simulink model "BugE_v0_40_MAS"  (R2015b)
settings: Solver=FixedStepDiscrete  StartTime=0.0  StopTime=inf  FixedStep=sample_time  RelTol=1e-3
values from neighbouring files (symbols this model uses):
  AB_diode_dV = 0.9    [main_sync.m]
  air_density = 1.225    [main_sync.m]
  bus_charger_Pmax = 1000    [main_sync.m]
  bus_load_Pmax_abs = 500    [main_sync.m]
  capInitVolt = capVmax*sqrt(capInitSoC)    [main_sync.m]
  cyc_kph = [cyc_kph(:,1), cyc_kph(:,2)*speed_max_limit/speed_max]    [main_sync.m]
  cyc_repeat = 0    [main_sync.m]
  ess1_init_soc = 1    [main_sync.m]
  ess1_soh = 1    [main_sync.m]
  ess2_init_soc = 1    [main_sync.m]
  ess2_soh = 1    [main_sync.m]
  ess3_init_soc = 1    [main_sync.m]
  ess3_soh = 1    [main_sync.m]
  ess4_init_soc = 1    [main_sync.m]
  ess4_soh = 1    [main_sync.m]
  ess5_init_soc = 1    [main_sync.m]
  ess5_soh = 1    [main_sync.m]
  gear_ratio = 6    [main_sync.m]
  loadpower = rawcsv(:,2)    [main_sync.m]
  loadtime = rawcsv(:,1)    [main_sync.m]
  lockSOCs = 0    [main_sync.m]
  max_brk_torque = 300    [main_sync.m]
  no_wheels = 3    [main_sync.m]
  period2 = max(loadtime)    [main_sync.m]
  PV_Pmax = 100    [main_sync.m]
  sample_time = 0.01    [main_sync.m]
  startup_seq_step_delay = 0.2    [main_sync.m]
  stop_option = 0    [main_sync.m]
  use_drive_cycle = 1    [main_sync.m]
  use_real_subs_loads = 1    [main_sync.m]
  vbus_max = 25    [main_sync.m]
  vbus_min = 17    [main_sync.m]
  vbus_safety_threshold = 2    [main_sync.m]
  vbus_threshold = 20    [main_sync.m]
  veh_CD = 0.35    [main_sync.m]
  veh_FA = 1.543    [main_sync.m]
  veh_gravity = 9.81*veh_mass    (= 1863.9)    [main_sync.m]
  veh_mass = 190    [main_sync.m]
  wh_1st_rrc = 0.02    [main_sync.m]
  wh_bearing_frc = 0.0015    [main_sync.m]
  wh_inertia = 0.0556    [main_sync.m]
  wh_radius = 0.508/2    (= 0.254)    [main_sync.m]
undefined symbols (not defined in the file or in its folder): capC, capR, cyc_acc, cyc_avg_time_samples, cyc_brk, cyc_grade, cyc_key, DCM_eff_factor_for_Vin, DCM_eff_for_Iout, DCM_Iout, DCM_Iout_max, DCM_Pin_noload, DCM_Pout_max, DCM_Vin, DCM_Vout, DiscIntNeverNeededParam, ess2_coulombic_eff, ess2_Ineg_max_SOC, ess2_Ineg_max_temp, ess2_Ipos_max_SOC, ess2_Ipos_max_temp, ess2_max_ah_cap, ess2_max_volts, ess2_min_volts, ess2_module_parallel, ess2_module_series, ess2_r_dis, ess2_soc, ess2_SOC_for_Ilimit, ess2_temp_for_Ilimit, ess2_temp_max, ess2_tmp, ess2_voc, ess3_coulombic_eff, ess3_max_ah_cap, ess3_module_parallel, ess3_module_series, ess3_r_dis, ess3_soc, ess3_tmp, ess3_voc, ess_coulombic_eff, ess_Ineg_max_SOC, ess_Ineg_max_temp, ess_Ipos_max_SOC, ess_Ipos_max_temp, ess_max_ah_cap, ess_max_volts, ess_min_volts, ess_module_parallel, ess_module_series, ess_nominal_volts, ess_r_dis, ess_soc, ess_SOC_for_Ilimit, ess_temp_for_Ilimit, ess_temp_max, ess_tmp, ess_voc, MC_eff1 ... (+17)
libraries: simulink x139, commfilt2 x1, simulink_extras x1
(part 7 of 7)

== system BugE_v0_40_MAS/Master Controller/Operating Mode Controller/State machine 0 std, 1 startup, 2 acc, 3 drv, 4 fault/pass10 ==
  I : Inport
  Logical Operator : Logic  Operator=NOT  AllPortsSameDT=off  OutDataTypeStr=boolean
  Logical Operator1 : Logic  Operator=NOT  AllPortsSameDT=off  OutDataTypeStr=boolean
  O : Outport
  wires:
  I/1 -> Logical Operator/1
  Logical Operator1/1 -> O/1
  Logical Operator/1 -> Logical Operator1/1

== system BugE_v0_40_MAS/Master Controller/Operating Mode Controller/State machine 0 std, 1 startup, 2 acc, 3 drv, 4 fault/pass2 ==
  I : Inport
  Logical Operator : Logic  Operator=NOT  AllPortsSameDT=off  OutDataTypeStr=boolean
  Logical Operator1 : Logic  Operator=NOT  AllPortsSameDT=off  OutDataTypeStr=boolean
  O : Outport
  wires:
  I/1 -> Logical Operator/1
  Logical Operator1/1 -> O/1
  Logical Operator/1 -> Logical Operator1/1

== system BugE_v0_40_MAS/Master Controller/Operating Mode Controller/State machine 0 std, 1 startup, 2 acc, 3 drv, 4 fault/pass3 ==
  I : Inport
  Logical Operator : Logic  Operator=NOT  AllPortsSameDT=off  OutDataTypeStr=boolean
  Logical Operator1 : Logic  Operator=NOT  AllPortsSameDT=off  OutDataTypeStr=boolean
  O : Outport
  wires:
  I/1 -> Logical Operator/1
  Logical Operator1/1 -> O/1
  Logical Operator/1 -> Logical Operator1/1

== system BugE_v0_40_MAS/Master Controller/Operating Mode Controller/State machine 0 std, 1 startup, 2 acc, 3 drv, 4 fault/pass4 ==
  I : Inport
  Logical Operator : Logic  Operator=NOT  AllPortsSameDT=off  OutDataTypeStr=boolean
  Logical Operator1 : Logic  Operator=NOT  AllPortsSameDT=off  OutDataTypeStr=boolean
  O : Outport
  wires:
  I/1 -> Logical Operator/1
  Logical Operator1/1 -> O/1
  Logical Operator/1 -> Logical Operator1/1

== system BugE_v0_40_MAS/Master Controller/Operating Mode Controller/State machine 0 std, 1 startup, 2 acc, 3 drv, 4 fault/pass5 ==
  I : Inport
  Logical Operator : Logic  Operator=NOT  AllPortsSameDT=off  OutDataTypeStr=boolean
  Logical Operator1 : Logic  Operator=NOT  AllPortsSameDT=off  OutDataTypeStr=boolean
  O : Outport
  wires:
  I/1 -> Logical Operator/1
  Logical Operator1/1 -> O/1
  Logical Operator/1 -> Logical Operator1/1

== system BugE_v0_40_MAS/Master Controller/Secondary Objectives/MB SOC balancing/Balancing type: 1: none, 2: P>0, 3: P<0 ==
  enable : Inport
  DCDC Iout (bus side) : Inport  Port=2
  enabled MODs : Inport  Port=3
  Data Type Conversion : DataTypeConversion
  Dead Zone +- 10E-3 : DeadZone  LowerValue=-10E-3  UpperValue=10E-3  SaturateOnIntegerOverflow=on
  Iout_total MB DCDC : Sum  Inputs=+
  Mux3 : Mux  Inputs=3
  P<0 : Gain  Gain=3  OutDataTypeStr=double
  P<0 balancing : simulink/Logic and Bit Operations/Compare To Constant  relop=<  const=0  OutDataTypeStr=boolean
  P=0 : Gain  OutDataTypeStr=double
  P>0 : Gain  Gain=2  OutDataTypeStr=double
  P>0 balancing : simulink/Logic and Bit Operations/Compare To Constant  relop=>  const=0  OutDataTypeStr=boolean
  Product : Product
  Saturation : Saturate  UpperLimit=3  LowerLimit=1
  and : Logic  AllPortsSameDT=off  OutDataTypeStr=boolean
  enable balancing : simulink/Logic and Bit Operations/Compare To Constant  relop=>=  const=2  OutDataTypeStr=boolean
  max : MinMax  Function=max
  no balancing : simulink/Logic and Bit Operations/Compare To Constant  relop===  const=0  OutDataTypeStr=boolean
  sum : Sum  Inputs=+
  type : Outport
  wires:
  no balancing/1 -> P=0/1
  DCDC Iout (bus side)/1 -> Iout_total MB DCDC/1
  Mux3/1 -> max/1
  Dead Zone +- 10E-3/1 -> no balancing/1, P<0 balancing/1, P>0 balancing/1
  P<0 balancing/1 -> P<0/1
  P>0/1 -> Mux3/2
  P<0/1 -> Mux3/3
  Iout_total MB DCDC/1 -> Dead Zone +- 10E-3/1
  P=0/1 -> Mux3/1
  P>0 balancing/1 -> P>0/1
  Product/1 -> Saturation/1
  max/1 -> Product/2
  enable/1 -> and/1
  Data Type Conversion/1 -> Product/1
  Saturation/1 -> type/1
  enabled MODs/1 -> sum/1
  sum/1 -> enable balancing/1
  enable balancing/1 -> and/2
  and/1 -> Data Type Conversion/1

== system BugE_v0_40_MAS/Master Controller/Secondary Objectives/MB SOC balancing/MB balancing through load distribution ==
  note: Pout MB DCDC
      | 1: none, 2: P>0, 3: P<0
  distribution type : Inport
  MOD's EN : Inport  Port=2
  MB SOCs : Inport  Port=3
  1/rel SOCs : Switch  Criteria=u2 > Threshold
  1/u : Math  Operator=reciprocal  RndMeth=Zero  SaturateOnIntegerOverflow=on
  >= eps : Saturate  UpperLimit=inf  LowerLimit=eps
  Constant1 : Constant  Value=3  SampleTime=sample_time
  Multiport Switch2 : MultiPortSwitch  SaturateOnIntegerOverflow=on
  SOCmax : MinMax  Function=max
  Scope : Scope
  "[1,10]" : Saturate  UpperLimit=10  LowerLimit=1
  "[eps,1]" : Saturate  UpperLimit=1  LowerLimit=eps
  bool2dbl : DataTypeConversion  OutDataTypeStr=double
  filtered SOCs (0 for dsbl'ed) : Product
  normalize (smallest = 1) : Product  Inputs=*/
  ones : Subsystem
  positive min : Subsystem
  relative SOCs : Product  Inputs=*/
  strengthen ratios : Math  Operator=pow  SaturateOnIntegerOverflow=on
  MB slope adj : Outport
  wires:
  distribution type/1 -> Multiport Switch2/1
  MOD's EN/1 -> bool2dbl/1
  bool2dbl/1 -> filtered SOCs (0 for dsbl'ed)/2
  MB SOCs/1 -> filtered SOCs (0 for dsbl'ed)/1
  "[eps,1]"/1 -> 1/u/1
  >= eps/1 -> relative SOCs/2
  SOCmax/1 -> >= eps/1
  filtered SOCs (0 for dsbl'ed)/1 -> 1/rel SOCs/2, SOCmax/1, relative SOCs/1, ones/1(I)
  1/u/1 -> 1/rel SOCs/1
  ones/1(O) -> 1/rel SOCs/3, Multiport Switch2/2
  relative SOCs/1 -> "[eps,1]"/1, Multiport Switch2/3
  Constant1/1 -> strengthen ratios/2
  1/rel SOCs/1 -> Multiport Switch2/4
  positive min/1(O) -> normalize (smallest = 1)/2
  Multiport Switch2/1 -> normalize (smallest = 1)/1, positive min/1(I)
  normalize (smallest = 1)/1 -> Scope/1, strengthen ratios/1
  strengthen ratios/1 -> "[1,10]"/1
  "[1,10]"/1 -> MB slope adj/1

== system BugE_v0_40_MAS/Master Controller/Secondary Objectives/Motor MBDCDC boost/ones ==
  I : Inport
  Bias : Bias  Bias=1
  Gain : Gain  Gain=0
  bool2dbl : DataTypeConversion  OutDataTypeStr=double
  O : Outport
  wires:
  Bias/1 -> O/1
  I/1 -> bool2dbl/1
  Gain/1 -> Bias/1
  bool2dbl/1 -> Gain/1

== system BugE_v0_40_MAS/Master Controller/System Health/Internally detected faults/20s moving avg (1//20 samples)1 ==
  In1 : Inport
  Counter Limited : simulink/Sources/Counter Limited  uplimit=19  tsamp=sample_time
  Triggered Subsystem : Subsystem  TreatAsAtomicUnit=on
  Out1 : Outport
  wires:
  Triggered Subsystem/1(Out1) -> Out1/1
  Counter Limited/1 -> Triggered Subsystem/Trigger
  In1/1 -> Triggered Subsystem/1(In1)

== system BugE_v0_40_MAS/Master Controller/System Health/Internally detected faults/20s moving avg (1//20 samples)3 ==
  In1 : Inport
  Counter Limited : simulink/Sources/Counter Limited  uplimit=19  tsamp=sample_time
  Triggered Subsystem : Subsystem  TreatAsAtomicUnit=on
  Out1 : Outport
  wires:
  Triggered Subsystem/1(Out1) -> Out1/1
  Counter Limited/1 -> Triggered Subsystem/Trigger
  In1/1 -> Triggered Subsystem/1(In1)

== system BugE_v0_40_MAS/Master Controller/System Health/Internally detected faults/40s moving avg (1//40 samples) ==
  In1 : Inport
  Counter Limited : simulink/Sources/Counter Limited  uplimit=39  tsamp=sample_time
  Triggered Subsystem : Subsystem  TreatAsAtomicUnit=on
  Out1 : Outport
  wires:
  Triggered Subsystem/1(Out1) -> Out1/1
  Counter Limited/1 -> Triggered Subsystem/Trigger
  In1/1 -> Triggered Subsystem/1(In1)

== system BugE_v0_40_MAS/Master Controller/System Health/Internally detected faults/diff >= 10% (or >1W for cmd=0) ==
  command : Inport
  result : Inport  Port=2
  !=0 : simulink/Logic and Bit Operations/Compare To Zero  relop=~=  OutDataTypeStr=boolean
  Constant : Constant  SampleTime=sample_time
  "Dead Zone [-0.1, 0.1]" : DeadZone  LowerValue=-0.1  UpperValue=0.1  SaturateOnIntegerOverflow=on
  "Dead Zone [-1, 1]" : DeadZone  LowerValue=-1  UpperValue=1  SaturateOnIntegerOverflow=on
  Divide : Product  Inputs=*/
  Subtract : Sum  Inputs=-+
  Switch avoid 0 div : Switch  Criteria=u2 > Threshold
  case where cmd=0 : Switch  Criteria=u2 > Threshold
  ~=0 : simulink/Logic and Bit Operations/Compare To Zero  relop=~=  OutDataTypeStr=boolean
  significant diff detected : Outport
  wires:
  Subtract/1 -> Divide/1
  command/1 -> !=0/1, Switch avoid 0 div/1, Subtract/2
  Divide/1 -> "Dead Zone [-0.1, 0.1]"/1
  ~=0/1 -> significant diff detected/1
  "Dead Zone [-0.1, 0.1]"/1 -> case where cmd=0/1
  Constant/1 -> Switch avoid 0 div/3
  Switch avoid 0 div/1 -> Divide/2
  !=0/1 -> case where cmd=0/2, Switch avoid 0 div/2
  result/1 -> "Dead Zone [-1, 1]"/1, Subtract/1
  "Dead Zone [-1, 1]"/1 -> case where cmd=0/3
  case where cmd=0/1 -> ~=0/1

== system BugE_v0_40_MAS/Master Controller/System Health/Internally detected faults/diff >= 10% (or >1W for cmd=0)1 ==
  command : Inport
  result : Inport  Port=2
  !=0 : simulink/Logic and Bit Operations/Compare To Zero  relop=~=  OutDataTypeStr=boolean
  Constant : Constant  SampleTime=sample_time
  "Dead Zone [-0.1, 0.1]" : DeadZone  LowerValue=-0.1  UpperValue=0.1  SaturateOnIntegerOverflow=on
  "Dead Zone [-1, 1]" : DeadZone  LowerValue=-1  UpperValue=1  SaturateOnIntegerOverflow=on
  Divide : Product  Inputs=*/
  Subtract : Sum  Inputs=-+
  Switch avoid 0 div : Switch  Criteria=u2 > Threshold
  case where cmd=0 : Switch  Criteria=u2 > Threshold
  ~=0 : simulink/Logic and Bit Operations/Compare To Zero  relop=~=  OutDataTypeStr=boolean
  significant diff detected : Outport
  wires:
  Subtract/1 -> Divide/1
  command/1 -> !=0/1, Switch avoid 0 div/1, Subtract/2
  Divide/1 -> "Dead Zone [-0.1, 0.1]"/1
  ~=0/1 -> significant diff detected/1
  "Dead Zone [-0.1, 0.1]"/1 -> case where cmd=0/1
  Constant/1 -> Switch avoid 0 div/3
  Switch avoid 0 div/1 -> Divide/2
  !=0/1 -> case where cmd=0/2, Switch avoid 0 div/2
  result/1 -> "Dead Zone [-1, 1]"/1, Subtract/1
  "Dead Zone [-1, 1]"/1 -> case where cmd=0/3
  case where cmd=0/1 -> ~=0/1

== system BugE_v0_40_MAS/Misc/Energy Calculations/E_battery_total/Battery losses ==
  Add : Sum  Inputs=5
  Unit Delay : UnitDelay  SampleTime=-1
  Out1 : Outport
  wires:
  [E_batt_loss2] -> Add/2
  [E_batt_loss1] -> Add/1
  Add/1 -> Out1/1
  [E_batt_loss4] -> Add/4
  Unit Delay/1 -> Add/5
  [E_batt_loss3] -> Add/3
  [E_batt_loss5] -> Unit Delay/1

== system BugE_v0_40_MAS/Misc/Energy Calculations/E_battery_total/Battery useful ==
  E_batt_useful : Sum  Inputs=5
  Unit Delay : UnitDelay  SampleTime=-1
  Out1 : Outport
  wires:
  [E_batt_useful3] -> E_batt_useful/3
  E_batt_useful/1 -> Out1/1
  [E_batt_useful5] -> Unit Delay/1
  [E_batt_useful1] -> E_batt_useful/1
  [E_batt_useful2] -> E_batt_useful/2
  [E_batt_useful4] -> E_batt_useful/4
  Unit Delay/1 -> E_batt_useful/5

== system BugE_v0_40_MAS/Auxiliaries (LV Grid)/AB (w// diode)/Calculate SOC/Resettable Integrator/Subsystem ==
  input : Inport
  IC : Inport  Port=2
  Enable : EnablePort  StatesWhenEnabling=reset
  Discrete-Time Integrator : DiscreteIntegrator  InitialConditionSource=external  InitialConditionSetting=State (most efficient)  SampleTime=sample_time  ICPrevOutput=DiscIntNeverNeededParam  ICPrevScaledInput=DiscIntNeverNeededParam
  Out1 : Outport
  wires:
  input/1 -> Discrete-Time Integrator/1
  IC/1 -> Discrete-Time Integrator/2
  Discrete-Time Integrator/1 -> Out1/1

== system BugE_v0_40_MAS/Auxiliaries (LV Grid)/AB (w// diode)/Calculate SOC/Resettable Integrator/Subsystem1 ==
  Enable : EnablePort
  Constant1 : Constant  SampleTime=sample_time
  Out1 : Outport  InitialOutput=0
  wires:
  Constant1/1 -> Out1/1

== system BugE_v0_40_MAS/Energy Storage (New Grid)/MB1/Calculate SOC/Resettable Integrator/Subsystem ==
  input : Inport
  IC : Inport  Port=2
  Enable : EnablePort  StatesWhenEnabling=reset
  Discrete-Time Integrator : DiscreteIntegrator  InitialConditionSource=external  InitialConditionSetting=State (most efficient)  SampleTime=sample_time  ICPrevOutput=DiscIntNeverNeededParam  ICPrevScaledInput=DiscIntNeverNeededParam
  Out1 : Outport
  wires:
  input/1 -> Discrete-Time Integrator/1
  IC/1 -> Discrete-Time Integrator/2
  Discrete-Time Integrator/1 -> Out1/1

== system BugE_v0_40_MAS/Energy Storage (New Grid)/MB1/Calculate SOC/Resettable Integrator/Subsystem1 ==
  Enable : EnablePort
  Constant1 : Constant  SampleTime=sample_time
  Out1 : Outport  InitialOutput=0
  wires:
  Constant1/1 -> Out1/1

== system BugE_v0_40_MAS/Energy Storage (New Grid)/MB2/Calculate SOC/Resettable Integrator/Subsystem ==
  input : Inport
  IC : Inport  Port=2
  Enable : EnablePort  StatesWhenEnabling=reset
  Discrete-Time Integrator : DiscreteIntegrator  InitialConditionSource=external  InitialConditionSetting=State (most efficient)  SampleTime=sample_time  ICPrevOutput=DiscIntNeverNeededParam  ICPrevScaledInput=DiscIntNeverNeededParam
  Out1 : Outport
  wires:
  input/1 -> Discrete-Time Integrator/1
  IC/1 -> Discrete-Time Integrator/2
  Discrete-Time Integrator/1 -> Out1/1

== system BugE_v0_40_MAS/Energy Storage (New Grid)/MB2/Calculate SOC/Resettable Integrator/Subsystem1 ==
  Enable : EnablePort
  Constant1 : Constant  SampleTime=sample_time
  Out1 : Outport  InitialOutput=0
  wires:
  Constant1/1 -> Out1/1

== system BugE_v0_40_MAS/Master Controller/Secondary Objectives/MB SOC balancing/MB balancing through load distribution/ones ==
  I : Inport
  Bias : Bias  Bias=1
  Gain : Gain  Gain=0
  O : Outport
  wires:
  Bias/1 -> O/1
  I/1 -> Gain/1
  Gain/1 -> Bias/1

== system BugE_v0_40_MAS/Master Controller/Secondary Objectives/MB SOC balancing/MB balancing through load distribution/positive min ==
  I : Inport
  " " : Terminator
  >0 Elem : Find  NumberOfInputDimensions=3  IndexMode=Zero-based  ShowOutputForNonzeroInputValues=on  SampleTime=sample_time
  Compare To Zero : simulink/Logic and Bit Operations/Compare To Zero  relop===  OutDataTypeStr=boolean
  Compare To Zero1 : simulink/Logic and Bit Operations/Compare To Zero  relop=>  OutDataTypeStr=boolean
  Merge : Merge
  Width : Width
  epsilon : Subsystem
  true min >0 : Subsystem
  O : Outport
  wires:
  >0 Elem/2 -> Width/1, true min >0/1(In1)
  I/1 -> >0 Elem/1
  >0 Elem/1 -> " "/1
  true min >0/1(Out1) -> Merge/2
  Merge/1 -> O/1
  Compare To Zero1/1 -> true min >0/Enable
  epsilon/1(Out1) -> Merge/1
  Compare To Zero/1 -> epsilon/Enable
  Width/1 -> Compare To Zero/1, Compare To Zero1/1

== system BugE_v0_40_MAS/Master Controller/System Health/Internally detected faults/20s moving avg (1//20 samples)1/Triggered Subsystem ==
  In1 : Inport
  Trigger : TriggerPort  TriggerType=falling
  1s moving avg : DiscreteFir  Coefficients=ones(1,1*(1/sample_time))/(1*(1/sample_time))
  Out1 : Outport
  wires:
  In1/1 -> 1s moving avg/1
  1s moving avg/1 -> Out1/1

== system BugE_v0_40_MAS/Master Controller/System Health/Internally detected faults/20s moving avg (1//20 samples)3/Triggered Subsystem ==
  In1 : Inport
  Trigger : TriggerPort  TriggerType=falling
  1s moving avg : DiscreteFir  Coefficients=ones(1,1*(1/sample_time))/(1*(1/sample_time))
  Out1 : Outport
  wires:
  In1/1 -> 1s moving avg/1
  1s moving avg/1 -> Out1/1

== system BugE_v0_40_MAS/Master Controller/System Health/Internally detected faults/40s moving avg (1//40 samples)/Triggered Subsystem ==
  In1 : Inport
  Trigger : TriggerPort  TriggerType=falling
  1s moving avg : DiscreteFir  Coefficients=ones(1,1*(1/sample_time))/(1*(1/sample_time))
  Out1 : Outport
  wires:
  In1/1 -> 1s moving avg/1
  1s moving avg/1 -> Out1/1

== system BugE_v0_40_MAS/Master Controller/Secondary Objectives/MB SOC balancing/MB balancing through load distribution/positive min/epsilon ==
  Enable : EnablePort
  eps : Constant  Value=0.0001  SampleTime=sample_time
  Out1 : Outport  InitialOutput=0.0001
  wires:
  eps/1 -> Out1/1

== system BugE_v0_40_MAS/Master Controller/Secondary Objectives/MB SOC balancing/MB balancing through load distribution/positive min/true min >0 ==
  In1 : Inport
  Enable : EnablePort
  SOCmin : MinMax
  Out1 : Outport  InitialOutput=1
  wires:
  In1/1 -> SOCmin/1
  SOCmin/1 -> Out1/1
